simulink library "Lib_Thermo_Enth2Temp_TMATS_new"  (R2015a)
settings: Solver=ode45  StartTime=0.0  StopTime=10.0  RelTol=1e-3
Description:
  | Thomas Modules
settings Model: Creator=jwchapm2  LastModifiedBy=jwhitfie
settings OptimizationCC: ExpressionDepthLimit=2147483647
settings DebuggingCC: UnderspecifiedInitializationDetection=Classic  MergeDetectMultiDrivingBlocksExec=none  SolverPrmCheckMsg=warning  StateNameClashWarn=warning

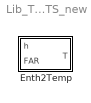
== system Lib_Thermo_Enth2Temp_TMATS_new ==
  Enth2Temp : Subsystem  mask(T-MATS: Enth2Temp Library Block){}
      mask help: This block emperically calculates temperature (T) from enthalpy (h) and fuel to air ratio (FAR).
      mask Help: web(which('Thermo_TMATS_Enth2Temp.html'),'-helpbrowser')

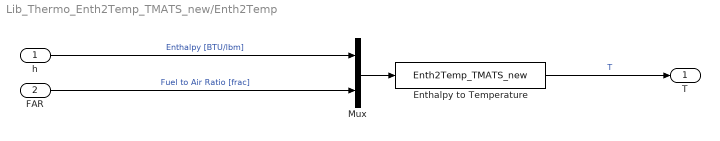
== system Lib_Thermo_Enth2Temp_TMATS_new/Enth2Temp ==
  h : Inport
  FAR : Inport  Port=2
  "Enthalpy to Temperature " : S-Function  FunctionName=Enth2Temp_TMATS_new  SFunctionModules='h2tc_TMATS'
  Mux : Mux  Inputs=2
  T : Outport
  wires:
  "Enthalpy to Temperature "/1 -> T/1  "T"
  Mux/1 -> "Enthalpy to Temperature "/1
  h/1 -> Mux/1  "Enthalpy [BTU/lbm]"
  FAR/1 -> Mux/2  "Fuel to Air Ratio [frac]"
